simulink model "px4demo_write_uorb_example"  (R2017b)
settings: Solver=FixedStepDiscrete  StartTime=0.0  StopTime=inf  RelTol=1e-3  EnableMultiTasking=on
InitFcn:
  | LAT = int32(10);
  | LON = int32(12);
  | ALT = int32(21);
libraries: pixhawk_slib_sensors_actuators x1
Description:
  | PX4 PSP Demo Model - uORB Write
  | 
  | This model demonstrates how one can write data to uORB topics
  | 
  | The uORB write block writes to the struct elements 'lat','lon' and 'timestamp'
  | to the GPS topic. The GPS block then outputs the same value we are writing
  | to by first advertising the GPS topic and then publishing data.
  | You can define whatever topic to write to and it's individual struct elements
  | 
  | 1) Define LAT, LON and TIME in the MATLAB work-space
  | 2) Run in external mode
  | 3) Tune values  LAT, LON and TIME and watch the values change in the display
  | from the output of the GPS block
  | 
  | NOTE: This model is to be demosntrated in external mode. An alternative to being able to
  | view these values without external mode is to modify this example to print the signals to
  |  the Nuttshell terminal using the print block
settings Model: SimulationMode=external  TunableVars=LAT,LON,ALT  TunableVarsStorageClass=Auto,Auto,Auto  TunableVarsTypeQualifier=,,  Creator=darenlee  LastModifiedBy=skuznick
settings SolverCC: PositivePriorityOrder=on
settings DataIOCC: LimitDataPoints=on  SaveFormat=StructureWithTime
settings OptimizationCC: DefaultParameterBehavior=Inlined  LifeSpan=1  MaxStackSize=64
settings DebuggingCC: AllowSymbolicDim=off  SFUnexpectedBacktrackingDiag=warning  SFNoUnconditionalDefaultTransitionDiag=warning  SFExecutionAtInitializationDiag=none
settings HardwareCC: ProdBitPerPointer=32  ProdBitPerSizeT=32  ProdBitPerPtrDiffT=32  ProdLargestAtomicInteger=Long  ProdLargestAtomicFloat=Double  ProdWordSize=32  ProdHWDeviceType=ARM Compatible->ARM Cortex
settings ModelReferenceCC: PropagateSignalLabelsOutOfModel=off
settings SFSimCC: MATLABDynamicMemAlloc=off
settings RTWCC: SystemTargetFile=ert.tlc  HardwareBoard=Pixhawk PX4  TemplateMakefile=ert_default_tmf  GenerateReport=on  Toolchain=Pixhawk Toolchain  BuildConfiguration=Faster Runs  IncludeHyperlinkInReport=on  LaunchReport=on  GenerateTraceInfo=on  GenerateTraceReport=on  GenerateTraceReportSl=on  GenerateTraceReportSf=on  GenerateTraceReportEml=on
settings CodeAppCC: IgnoreCustomStorageClasses=off  StateflowObjectComments=on
settings ERTTargetCC: MultiwordLength=2048  ExtMode=on  ExtModeTransport=1  ExtModeMexFile=ext_serial_win32_comm  ExtModeMexArgs=1 7 115200  ERTCustomFileTemplate=px4_codertarget_file_process.tlc  ConvertIfToSwitch=off  SuppressUnreachableDefaultCases=off
settings ConfigComp: CovMetricSettings=dw  CovHtmlReporting=on  CovSaveCumulativeToWorkspaceVar=on  CovSaveSingleToWorkspaceVar=on  CovExternalEMLEnable=off

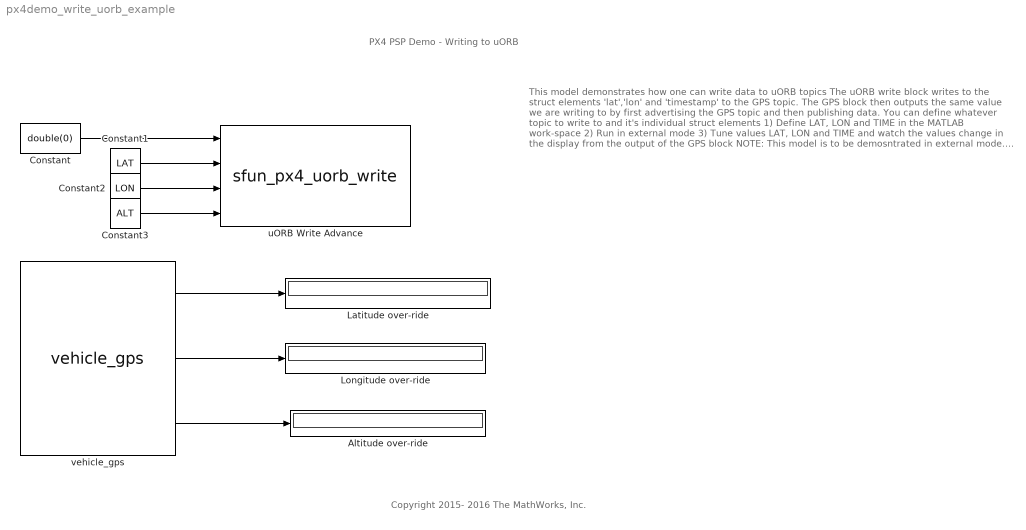
== system px4demo_write_uorb_example ==
  note: This model demonstrates how one can write data to uORB topics
      |
      | The uORB write block writes to the struct elements 'lat','lon' and 'timestamp'
      | to the GPS topic. The GPS block then outputs the same value we are writing
      | to by first advertising the GPS topic and then publishing data.
      | You can define whatever topic to write to and it's individual struct elements
      |
      | 1) Define LAT, LON and TIME in the MATLAB work-space
      | 2) Run in external mode
      | 3) Tune values LAT, LON and TIME and watch the values change in the display
      | from the output of the GPS block
      |
      | NOTE: This model is to be demosntrated in external mode. An alternative to being able to
      | view these values without external mode is to modify this example to print the signals to
      | the Nuttshell terminal using the print block
  note: PX4 PSP Demo - Writing to uORB
  note: Copyright 2015- 2016 The MathWorks, Inc.
  Altitude over-ride : Display
  Constant : Constant  Value=double(0)
  Constant1 : Constant  Value=LAT  OutDataTypeStr=int32  SampleTime=0.1
  Constant2 : Constant  Value=LON  OutDataTypeStr=int32  SampleTime=0.1
  Constant3 : Constant  Value=ALT  OutDataTypeStr=int32  SampleTime=0.1
  Latitude over-ride : Display
  Longitude over-ride : Display
  uORB Write Advance : S-Function  FunctionName=sfun_px4_uorb_write  Parameters=Ts, uORB_Topic_str, int32(uORB_Struct_DT), int32(BlockInputCount),char(uORB_StructParams),int32(uORB_PortSizes),uint32(uORB_AdvtQueue),uint32(MsgSizeOf)  SFunctionDeploymentMode=off  EnableBusSupport=off  SFcnStateName=uorb_msg  mask{Ts=0, uORB_AdvtQueue=on, uORB_FieldEnabledArr=0  0  0  1  0  0  0  0  0  0  0, uORB_Topic_str=0, uORB_Struct_DT=[1  1  1  1  1], BlockInputCount=5, uORB_StructParams=["voltage_v","voltage_filtered_v","current_a","current_filtered_a","remaining"], uORB_PortSizes=[1  1  1  1], MsgSizeOf=0, MW_update=true}
      mask help:
      | uORB Write Output Block
      |
      | Publishes to a user provided named tropic structure.
      mask init:
      | % A structure of data can be stored in the block UserData
      | maskData = get_param(gcb,'UserData');
      | % Block Param formatted string
      | if isfield(maskData,'uORBMsg')
      |     uORB_Topic_str = maskData.uORBMsg;
      | else
      |     uORB_Topic_str = '<unformatted_placeholder_param>';
      | end
      | 
      | if isfield(maskData,'SFuncParam_DTArr')
      |     uORB_Struct_DT = maskData.SFuncParam_DTArr;
      | else
      |     uORB_Struct_DT = [1];
      | end
      | 
      | if isfield(maskData,'SFuncParam_InputCount')
      |     BlockInputCount = maskData.SFuncParam_InputCount;
      | else
      |     BlockInputCount = '["<unformatted_placeholder_param>"]';
      | end
      | 
      | % NumParams
      | if isfield(maskData,'SFuncParam_PortSizes')
      |     uORB_PortSizes =  maskData.SFuncParam_PortSizes;
      | else
      |     uORB_PortSizes = 1;
      | end
      | 
      | if isfield(maskData,'FieldEnabled')
      |     uORB_FieldEnabledArr = maskData.FieldEnabled;
      | else
      |     uORB_FieldEnabledArr = [true];
      | end
      | 
      | if isfield(maskData,'SFuncParam_TLCStr')
      |     uORB_StructParams = maskData.SFuncParam_TLCStr;
      | else
      |     uORB_StructParams = [];
      | end
      | 
      | % Sample-time
      | if isfield(maskData,'Ts') 
      |     try
      |         Ts = evalin('base',maskData.Ts);
      |     catch
      |         Ts = -1;
      |     end
      | else
      |     Ts = -1;
      | end
      | 
      | % Advt Queue
      | if isfield(maskData,'AdvtQueue') 
      |     try
      |         uORB_AdvtQueue = evalin('base',maskData.AdvtQueue);
      |     catch
      |         uORB_AdvtQueue = 0;
      |     end
      | else
      |     uORB_AdvtQueue = 0;
      | end
      | 
      | % Force parameter data type
      | Ts = double(Ts);
      | uORB_FieldEnabledArr = boolean(uORB_FieldEnabledArr);
      | uORB_Topic_str = char(uORB_Topic_str);
      | uORB_Struct_DT = int32(uORB_Struct_DT);
      | BlockInputCount = int32(BlockInputCount);
      | uORB_StructParams = char(uORB_StructParams);
      | uORB_PortSizes = int32(uORB_PortSizes);
      | uORB_AdvtQueue = uint32(uORB_AdvtQueue);
      | 
      | % Get the size of the msg struct
      | MsgSizeOf = 0;
      | path_to_msg = fullfile(codertarget.pixhawk.internal.getPX4RootDir,'Firmware','msg',[uORB_Topic_str '.msg' ]);
      | [~,~,MsgSizeOf] = codertarget.pixhawk.blocks.Block_Callbacks.uORB.uORB_ParseMsgFile(path_to_msg);
      | %debug: fprintf('Byte Value = %d \n',MsgSizeOf);
      settings: OpenFcn=codertarget.pixhawk.blocks.Block_Callbacks.uORB.ParamUpdateMaskDialog_uORB_Write(gcbh);  SFcnIsStateOwnerBlock=on
      mask Display:
      | maskData = get_param(gcb,'UserData');
      | fprintf('uORB Write \n Topic: %s ',maskData.uORBMsg)
      | 
      | InputStrSrc = maskData.SFuncParam_TLCStr;
      | 
      | [idx_start,idx_end] = regexp(InputStrSrc,'\"([^\"]*)\"');
      | 
      | NumOfInputs = length(idx_start);
      | 
      | for idx = 1:NumOfInputs
      |     PortName = InputStrSrc(idx_start(idx):idx_end(idx));
      |     PortName = strrep(PortName,'"','');
      |     port_label('input',idx,PortName);
      | end
  vehicle_gps : pixhawk_slib_sensors_actuators/vehicle_gps  sampletime=1  show_alt=on  show_ts_gps=off  show_vel=off  show_fixtype=off  show_numsat=off
      settings: SourceProductName=Pixhawk Target Blocks
  wires:
  vehicle_gps/1 -> Latitude over-ride/1
  vehicle_gps/2 -> Longitude over-ride/1
  vehicle_gps/3 -> Altitude over-ride/1
  Constant3/1 -> uORB Write Advance/4
  Constant2/1 -> uORB Write Advance/3
  Constant1/1 -> uORB Write Advance/2
  Constant/1 -> uORB Write Advance/1
